simulink library "Window"  (R2018b)
settings: Solver=ode45  StartTime=0.0  StopTime=10.0  RelTol=1e-3  EnableMultiTasking=on
libraries: carnot x2, simulink_extras x2
settings Model: Creator=bernd.hafner  LastModifiedBy=drhf
settings DataIOCC: LimitDataPoints=on  SaveFormat=Array  SignalLoggingSaveFormat=ModelDataLogs
settings OptimizationCC: ExpressionDepthLimit=2147483647  LifeSpan=inf
settings DebuggingCC: UnderspecifiedInitializationDetection=Classic  MergeDetectMultiDrivingBlocksExec=none  SolverPrmCheckMsg=warning  FcnCallInpInsideContextMsg=warning  StateNameClashWarn=warning  SFUnexpectedBacktrackingDiag=warning  SFNoUnconditionalDefaultTransitionDiag=warning  SFExecutionAtInitializationDiag=none
settings HardwareCC: ProdBitPerPointer=32  ProdBitPerSizeT=32  ProdBitPerPtrDiffT=32  ProdLargestAtomicFloat=None  ProdIntDivRoundTo=Undefined  ProdEndianess=Unspecified  ProdWordSize=32  ProdHWDeviceType=32-bit Generic
settings ModelReferenceCC: PropagateSignalLabelsOutOfModel=off
settings SFSimCC: SimUseLocalCustomCode=off
settings RTWCC: RTWUseLocalCustomCode=off
settings CodeAppCC: StateflowObjectComments=on
settings GRTTargetCC: TargetLangStandard=C89/C90 (ANSI)  GeneratePreprocessorConditionals=Disable all  CombineOutputUpdateFcns=off  GRTInterface=on
settings ConfigComp: CovMetricSettings=dw  CovHtmlReporting=on  CovSaveCumulativeToWorkspaceVar=on  CovSaveSingleToWorkspaceVar=on  CovExternalEMLEnable=off

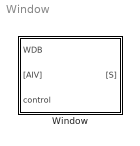
== system Window ==
  Window : Subsystem  mask(window){pos=0, windowsize=[1 1], frame=0.1, Ug=1.8, gvalue=0.6, tauzero=0.6*0.95, numpanes=2, d=[0.004 0.004], rho=[2500 2500], cp=[1008  1008], t0=20, misc=[0.2 0.1 1 1], shad_type=No shading, type_glazing=double glazing normal, tau_shad=0.01, bli_a=0.05, bli_b=1, bli_c=0.05, bli_d=0.05, bli_alpha=90, bli_refl=0.2}
      mask prompts: pos "azimut (0=south, east = -90)"; windowsize "size of window [m] [height width]"; frame "part of frame of the surface (0..1)"; Ug "heat transfer coefficient (U-value) [W/m²K]"; gvalue "Solar heat gain coefficient (SHGC) [0..1]"; tauzero "Primary solar heat gain (MUST be <= SHGC)"; numpanes "number of glass panes [1..4]"; d "thickness of glass panes [m] (vector with one element per pane)"; rho "density of glass [kg/m³] (vector with one element per pane)"; cp "capacity of glass [J/(kg*K)] (vector with one element per pane)"; t0 "initial temperature [°C]"; misc "[reflection_ground absorption_out emission_out emission_in]"; shad_type "shading type [no Shading/exterior/interior]"; type_glazing "glazing type"; tau_shad "solar transmittance of shading element [0..1]"; bli_a "a  Depth of blind blades [m]"; bli_b "b heigth of blind blades [m]"; bli_c "c distance of "b" to back end of blind blade [m]"; bli_d "d offset between blind blades [m]"; bli_refl "optical reflectance of blind surface [0..1]"
      mask help:
      | The window model evaluates the solar heat gain coefficient and the u-value to build up a two node model. The solar heat gain coefficient (SHGC) is the fraction of solar radiation admitted through a window, door, or skylight -- either transmitted directly and/or absorbed, and subsequently released as heat inside a home. The lower the SHGC, the less solar heat it transmits and the greater its shading ability.  The solar heat gain coefficient (SHGC) consists of two components:
      | + Primary solar heat gain: the solar heat directly transmitted through a glass in its original solar radiation form.
      | + Secondary solar heat gain: the solar heat absorbed by a glass and further transferred to the indoor space as heat by conduction, connection and radiation.
      | Control input [0..1] = fraction of shading (0 - no shading,   1 - full shading)
      mask init:
      | % Geometry
      | h = windowsize(1);
      | w = windowsize(2);
      | windowsurface = h*w;
      | if length(pos) == 1
      |     pos = [90  pos 0]; % pos is [inclination azimut rotation]
      | end
      | 
      | % Optics
      | reflectground = max(0, min(1, misc(1)));
      | absorption_out = max(0, min(1, misc(2)));
      | emission_out = max(0, min(1, misc(3)));
      | emission_in = max(0, min(1, misc(4)));
      | 
      | % Thermal
      | R_norm_in = 1/8;     % h_int = 8 W/m²/K set according to ISO
      | R_norm_out = 1/25;   % h_out = 25 W/m²/K set according to ISO
      | Rwin = 1/Ug - R_norm_in - R_norm_out;
      | % C = sum(cp.*rho.*d.^2); % old equation
      | C = sum(cp.*rho.*d); % corrected equation, hf 29nov2017
      | timeconst = Rwin*C/2;
      mask Help: web(fullfile(path_carnot('help'),'WindowWithShading.html'),'-helpbrowser')
      mask TypeOptions shad_type: alfa_window_in/shad_type
      mask Callback shad_type:
      | switch get_param(gcb,'shad_type')
      |         case 'No shading' % nr. 1 no shading
      |             set_param(gcb,'MaskVisibilities',{'on','on','on','on','on','on','on','on','on','on','on','on','on','off','off','off','off','off','off','off','off'});
      |         case 'Exterior Screen' % nr. 2 external screen
      |             set_param(gcb,'MaskVisibilities',{'on','on','on','on','on','on','on','on','on','on','on','on','on','off','on','off','off','off','off','off','off'});
      |         case 'Interior Screen' % nr. 3 Interior Screen
      |             set_param(gcb,'MaskVisibilities',{'on','on','on','on','on','on','on','on','on','on','on','on','on','on','on','off','off','off','off','off','off'});
      |         case 'Venetian Blind' % nr. 4 venetian blind
      |             set_param(gcb,'MaskVisibilities',{'on','on','on','on','on','on','on','on','on','on','on','on','on','off','off','on','on','on','on','on','on'});
      |     end
      mask TypeOptions type_glazing: alfa_window_in/type_glazing
      mask TypeOptions tau_shad: alfa_window_in/tau_shad
      mask TypeOptions bli_a: alfa_window_in/bli_a
      mask TypeOptions bli_b: alfa_window_in/bli_b
      mask TypeOptions bli_c: alfa_window_in/bli_c
      mask TypeOptions bli_d: alfa_window_in/bli_d
      mask TypeOptions bli_alpha: alfa_window_in/bli_alpha
      mask TypeOptions bli_refl: alfa_window_in/bli_refl

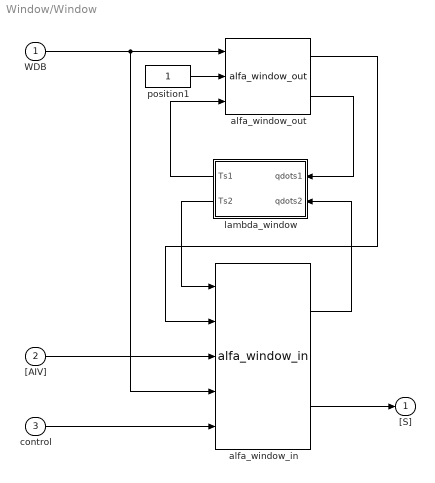
== system Window/Window ==
  WDB : Inport
  "[AIV]" : Inport  Port=2
  control : Inport  Port=3
  alfa_window_in : carnot/Basic/Heat_Transfer/alfa_window_in  type_glazing=double glazing normal  gvalue=gvalue  tauzero=tauzero  emission_in=misc(4)  wallsurface=windowsurface  frame=frame  numlayer=numpanes  shad_type=No shading  tau_shad=tau_shad  bli_a=bli_a  bli_b=bli_b  bli_c=bli_c  bli_d=bli_d  bli_alpha=bli_alpha  bli_refl=bli_refl
      settings: SourceProductName=Carnot
  alfa_window_out : carnot/Basic/Heat_Transfer/alfa_window_out  pos=pos  absorption_out=absorption_out  emission_out=emission_out  frame=frame
      settings: SourceProductName=Carnot
  lambda_window : Subsystem  mask(LAMBDA){}
      mask help:
      | Heat conduction through a transparent component (window).
      |
      | qdots1	: specific heat flow vertical on surface 1, W/m²
      | qdots2	: specific heat flow vertical on surface 2, W/m²
      | Ts1	: temperature of surface 1, °C
      | Ts2	: temperature of surface 2, °C
      |
      | NOTE CONVENTION for INPUT NUMBER:
      | "1"	  indoor surface of an outer window OR
      | 	  surface "a" of an inner window OR
      |  	  surface "f" of a glass floor
      |
      | "2"	  outdoor surface of a window OR
      | 	  surface "b" of an inner window OR
      |  	  surface "c" of a glass ceiling
  position1 : Constant
  "[S]" : Outport
  wires:
  position1/1 -> alfa_window_out/2
  control/1 -> alfa_window_in/5
  alfa_window_out/1 -> alfa_window_in/2
  alfa_window_out/2 -> lambda_window/1(qdots1)
  alfa_window_in/2 -> "[S]"/1
  alfa_window_in/1 -> lambda_window/2(qdots2)
  "[AIV]"/1 -> alfa_window_in/3
  WDB/1 -> alfa_window_out/1, alfa_window_in/4
  lambda_window/1(Ts1) -> alfa_window_out/3
  lambda_window/2(Ts2) -> alfa_window_in/1

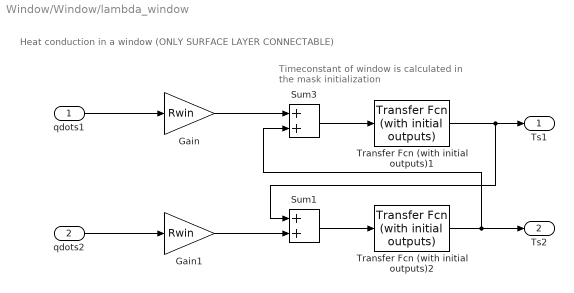
== system Window/Window/lambda_window ==
  note: Heat conduction in a window (ONLY SURFACE LAYER CONNECTABLE)
  note: Timeconstant of window is calculated
      | in the mask initialization
  qdots1 : Inport
  qdots2 : Inport  Port=2
  Gain : Gain  Gain=Rwin
  Gain1 : Gain  Gain=Rwin
  Sum1 : Sum  SaturateOnIntegerOverflow=on  InputSameDT=on  OutDataTypeStr=Inherit: Same as first input
  Sum3 : Sum  SaturateOnIntegerOverflow=on  InputSameDT=on  OutDataTypeStr=Inherit: Same as first input
  Transfer Fcn (with initial outputs)1 : simulink_extras/Additional Linear/Transfer Fcn (with initial outputs)  N=[1]  D=[timeconst 1]  Y0=t0  U0=t0
  Transfer Fcn (with initial outputs)2 : simulink_extras/Additional Linear/Transfer Fcn (with initial outputs)  N=[1]  D=[timeconst 1]  Y0=t0  U0=t0
  Ts1 : Outport
  Ts2 : Outport  Port=2
  wires:
  Transfer Fcn (with initial outputs)2/1 -> Ts2/1, Sum3/2
  Transfer Fcn (with initial outputs)1/1 -> Sum1/1, Ts1/1
  qdots1/1 -> Gain/1
  Sum3/1 -> Transfer Fcn (with initial outputs)1/1
  qdots2/1 -> Gain1/1
  Sum1/1 -> Transfer Fcn (with initial outputs)2/1
  Gain/1 -> Sum3/1
  Gain1/1 -> Sum1/2
